simulink model "servo_harness"  (R2021a)
settings: Solver=FixedStepAuto  StartTime=0.0  StopTime=5  FixedStep=0.001  RelTol=1e-3
undefined symbols (not defined in the file): sigbuilder_block
settings Model: DataDictionary=servo.sldd  Creator=Nabil  LastModifiedBy=Nabil

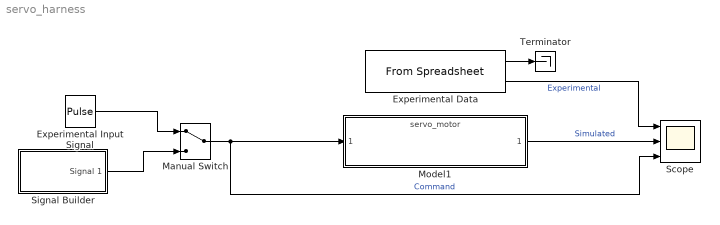
== system servo_harness ==
  Experimental Data : FromSpreadsheet  FileName=data3.csv  SheetName=data3
  Experimental Input Signal : DiscretePulseGenerator  PulseType=Time based  Amplitude=90  PulseWidth=50  PhaseDelay=0.615  VectorParams1D=off
  Manual Switch : ManualSwitch
  Model1 : ModelReference  ModelNameDialog=servo_motor.slx  SimulationMode=Normal  ModelReferenceVersion=8.14
  Scope : Scope  NumInputPorts=3
  Signal Builder : Subsystem  Tag=STV Subsys  LoadFcn=sigbuilder_block('load');  StartFcn=sigbuilder_block('start');  StopFcn=sigbuilder_block('stop');  ClipboardFcn=sigbuilder_block('clipboard');  mask(Sigbuilder block){tuvar=[0:10]}
      mask help: Simulink:masks:SigbuilderBlock_MD
      mask init:
      | if ~strcmp(get_param(bdroot(gcbh),'SimulationStatus'),'stopped') tuvar = sigbuilder_block('maskInit'); end
      settings: CopyFcn=sigbuilder_block('copy');  DeleteFcn=sigbuilder_block('delete');  ModelCloseFcn=sigbuilder_block('modelClose');  PreSaveFcn=sigbuilder_block('preSave');  PauseFcn=sigbuilder_block('pause');  ContinueFcn=sigbuilder_block('continue');  NameChangeFcn=sigbuilder_block('namechange');  OpenFcn=sigbuilder_block('open',[437.6 199.2 550.4 400 ]);  CloseFcn=sigbuilder_block('close');
      mask Display: plot(0, 0, 100, 100,[2, 2, 32, 32, 2], [68, 8, 8, 68, 68],[32, 2], [38, 38], [32, 19, 2],[53, 60, 44], [32, 17, 17, 2],[16, 16, 31, 31]);txt = getActiveGroup(gcbh);text(2, 100, txt,'verticalAlignment', 'top');
  Terminator : Terminator
  wires:
  Model1/1 -> Scope/2  "Simulated"
  Experimental Input Signal/1 -> Manual Switch/1
  Manual Switch/1 -> Scope/3, Model1/1  "Command"
  Signal Builder/1(Signal 1) -> Manual Switch/2
  Experimental Data/2 -> Scope/1  "Experimental"
  Experimental Data/1 -> Terminator/1

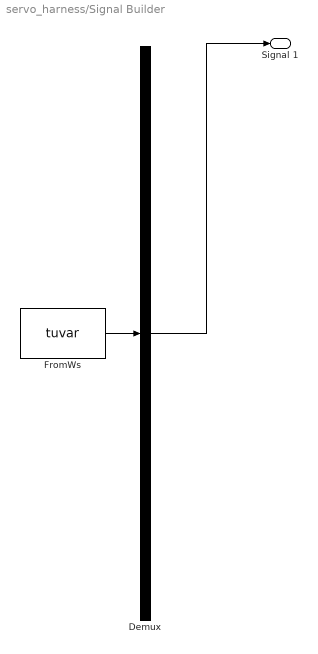
== system servo_harness/Signal Builder ==
  Demux : Demux  Tag=STV Demux  Outputs=1
      settings: DisplayOption=none
  FromWs : FromWorkspace  Tag=STV FromWs  VariableName=tuvar
      SigBuilderData=|
      | common.afterFinalStr = 'Extrapolate'
      | common.sampleTime = 0
      | dataSet.timeRange = [0 10]
      | dataSet.name = 'Group 1'
      | sbobj.Groups.Name = 'Group 1'
      | sbobj.Groups.Signals.Name = 'Signal 1'
      | sbobj.Groups.Signals.XData = [0 2.48 4.62 4.94 4.94 7.28 7.28 7.9 10]
      | sbobj.Groups.Signals.YData = [-0.01 8.8 2.2 0.5 4.5 15 2.5 5.4 0]
  Signal 1 : Outport  Tag=STV Outport
  wires:
  Demux/1 -> Signal 1/1
  FromWs/1 -> Demux/1
